simulink library "calculateReelOutRudderAngle"  (R2018a)
settings: Solver=VariableStepAuto  StartTime=0.0  StopTime=10.0  RelTol=1e-3
undefined symbols (not defined in the file): ctrl, env, plant
libraries: lowLevel x1, controllerComponents x1, dspsigops x1
settings Model: Creator=mitch  LastModifiedBy=mitch

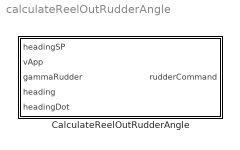
== system calculateReelOutRudderAngle ==
  CalculateReelOutRudderAngle : Subsystem

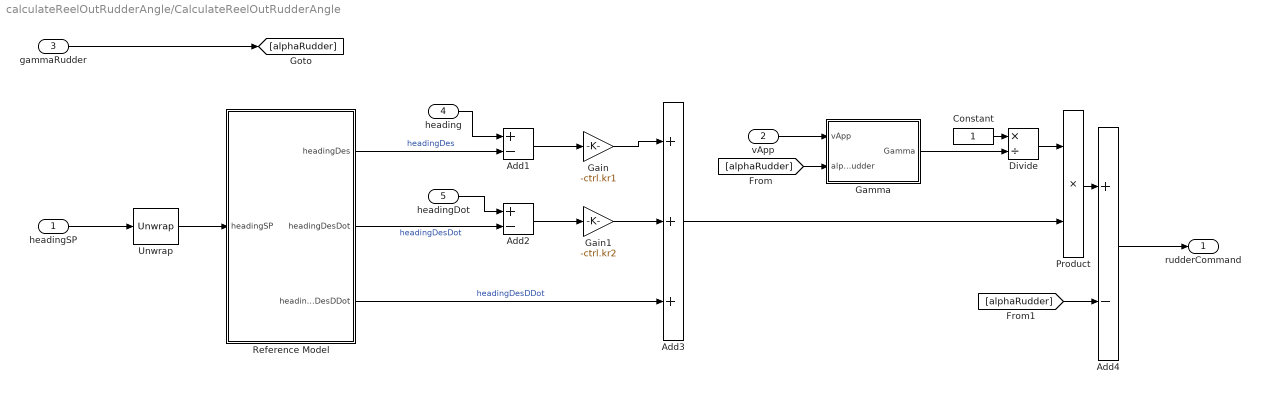
== system calculateReelOutRudderAngle/CalculateReelOutRudderAngle ==
  headingSP : Inport
  vApp : Inport  Port=2
  gammaRudder : Inport  Port=3
  heading : Inport  Port=4
  headingDot : Inport  Port=5
  Add1 : Sum  Inputs=+-
  Add2 : Sum  Inputs=+-
  Add3 : Sum  Inputs=+++
  Add4 : Sum  Inputs=+-
  Constant : Constant
  Divide : Product  Inputs=*/
  Gain : Gain  Gain=-ctrl.kr1
  Gain1 : Gain  Gain=-ctrl.kr2
  Gamma : Subsystem
  Product : Product
  Reference Model : Subsystem
  Unwrap : dspsigops/Unwrap  tol=pi  InputProcessing=Columns as channels (frame based)  running=off
  rudderCommand : Outport
  wires:
  Add3/1 -> Product/2
  gammaRudder/1 -> [alphaRudder]
  Add4/1 -> rudderCommand/1
  Unwrap/1 -> Reference Model/1(headingSP)
  Constant/1 -> Divide/1
  Add1/1 -> Gain/1
  heading/1 -> Add1/1
  Divide/1 -> Product/1
  Product/1 -> Add4/1
  [alphaRudder] -> Add4/2
  Gamma/1(Gamma) -> Divide/2
  Add2/1 -> Gain1/1
  Reference Model/1(headingDes) -> Add1/2  "headingDes"
  Gain1/1 -> Add3/2
  Reference Model/2(headingDesDot) -> Add2/2  "headingDesDot"
  [alphaRudder] -> Gamma/2(alphaRudder)
  vApp/1 -> Gamma/1(vApp)
  Reference Model/3(headingDesDDot) -> Add3/3  "headingDesDDot"
  headingSP/1 -> Unwrap/1
  Gain/1 -> Add3/1
  headingDot/1 -> Add2/1

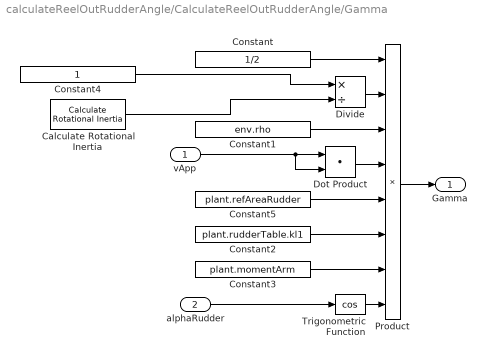
== system calculateReelOutRudderAngle/CalculateReelOutRudderAngle/Gamma ==
  vApp : Inport
  alphaRudder : Inport  Port=2
  Calculate Rotational Inertia : lowLevel/Calculate Rotational Inertia
  Constant : Constant  Value=1/2
  Constant1 : Constant  Value=env.rho
  Constant2 : Constant  Value=plant.rudderTable.kl1
  Constant3 : Constant  Value=plant.momentArm
  Constant4 : Constant
  Constant5 : Constant  Value=plant.refAreaRudder
  Divide : Product  Inputs=*/
  Dot Product : DotProduct  InputSameDT=on  OutDataTypeStr=Inherit: Inherit via internal rule
  Product : Product  Inputs=8
  Trigonometric Function : Trigonometry  Operator=cos
  Gamma : Outport
  wires:
  Constant3/1 -> Product/7
  Constant5/1 -> Product/5
  Constant/1 -> Product/1
  Constant2/1 -> Product/6
  Constant1/1 -> Product/3
  Dot Product/1 -> Product/4
  vApp/1 -> Dot Product/2, Dot Product/1
  alphaRudder/1 -> Trigonometric Function/1
  Trigonometric Function/1 -> Product/8
  Product/1 -> Gamma/1
  Divide/1 -> Product/2
  Calculate Rotational Inertia/1 -> Divide/2
  Constant4/1 -> Divide/1

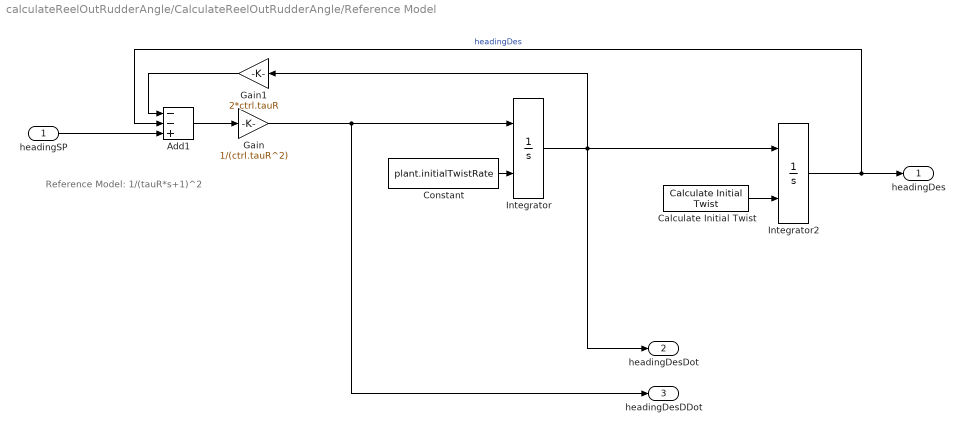
== system calculateReelOutRudderAngle/CalculateReelOutRudderAngle/Reference Model ==
  note: Reference Model:
      | 1/(tauR*s+1)^2
  headingSP : Inport
  Add1 : Sum  Inputs=--+
  Calculate Initial Twist : controllerComponents/Calculate Initial Twist
  Constant : Constant  Value=plant.initialTwistRate
  Gain : Gain  Gain=1/(ctrl.tauR^2)
  Gain1 : Gain  Gain=2*ctrl.tauR
  Integrator : Integrator  InitialConditionSource=external
  Integrator2 : Integrator  InitialConditionSource=external  InitialCondition=plant.initialTwist
  headingDes : Outport
  headingDesDot : Outport  Port=2
  headingDesDDot : Outport  Port=3
  wires:
  Gain/1 -> headingDesDDot/1, Integrator/1
  Integrator/1 -> Integrator2/1, headingDesDot/1, Gain1/1
  Add1/1 -> Gain/1
  Integrator2/1 -> Add1/2, headingDes/1  "headingDes"
  headingSP/1 -> Add1/3
  Gain1/1 -> Add1/1
  Calculate Initial Twist/1 -> Integrator2/2
  Constant/1 -> Integrator/2
